simulink model "RobotSim"  (R2013a)
settings: Solver=ode45  StartTime=0.0  StopTime=5.00  FixedStep=0.01  MaxStep=0.02  MinStep=1e-16  RelTol=1e-3
values from neighbouring files (symbols this model uses):
  alpha_p = constr.alpha_p    [ConstrGui.m]    (also in RunSim.m = constrData(1).alpha_p; optimiseConstraint.m = [alpha_ends(:,1:2), alpha_p_infix, alpha_ends(:,3:4)])
  ground = [-realmax, 0 ... (first row only)    [RunSim.m]    (also in runSim2.m)
  nom_torque = [constrData.th_base; u_nom]    [RunSim.m]
  org = endSwingFoot(q(:,end),org)    [RunSim.m]    (also in runSim2.m = [0, 0])
  q_0 = q_0'    [RunSim.m]
  qd_0 = qd_0'    [RunSim.m]    (also in periodic_qd0.m = [2*pi; pi])
  theta_p = constr.theta_p    [ConstrGui.m]    (also in RunSim.m = constrData(1).theta_p; optimiseConstraint.m = linspace(theta_ends(1), theta_ends(2), degree+1))
settings Model: CovHTMLOptions=-sRT=1 -aTS=1 -bRG=1 -bTC=1 -hTR=0 -nFC=0 -scm=1 -bcm=1 -xEv=0  Creator=yak  LastModifiedBy=yak
settings SolverCC: MaxConsecutiveMinStep=10
settings DataIOCC: LimitDataPoints=off  OutputOption=SpecifiedOutputTimes  OutputTimes=0:0.01:(timeleft-0.01)
settings DebuggingCC: DiscreteInheritContinuousMsg=none  MultiTaskDSMMsg=warning  MultiTaskCondExecSysMsg=none  FcnCallInpInsideContextMsg=EnableAllAsWarning  StrictBusMsg=None
settings RTWCC: IncludeERTFirstTime=on

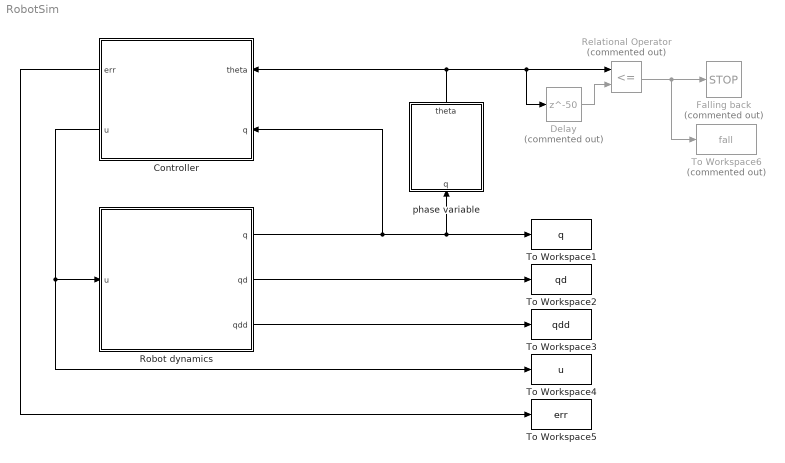
== system RobotSim ==
  Controller : Subsystem
  Delay : Delay  Commented=on  DelayLength=50  InitialCondition=-100  SampleTime=0.01
  Falling back : Stop  Commented=on
  Relational Operator : RelationalOperator  Commented=on  Operator=<=  OutDataTypeStr=boolean  ZeroCross=off
  Robot dynamics : Subsystem
  To Workspace1 : ToWorkspace  VariableName=q  SampleTime=-1
  To Workspace2 : ToWorkspace  VariableName=qd  SampleTime=-1
  To Workspace3 : ToWorkspace  VariableName=qdd  SampleTime=-1
  To Workspace4 : ToWorkspace  VariableName=u  SampleTime=-1
  To Workspace5 : ToWorkspace  VariableName=err  SampleTime=-1
  To Workspace6 : ToWorkspace  Commented=on  VariableName=fall  SampleTime=-1
      settings: MaxDataPoints=1
  phase variable : MATLAB Function  TreatAsAtomicUnit=on
  wires:
  Controller/2(u) -> Robot dynamics/1(u), To Workspace4/1
  Robot dynamics/1(q) -> Controller/2(q), To Workspace1/1, phase variable/1(q)
  Relational Operator/1 -> To Workspace6/1, Falling back/1
  phase variable/1(theta) -> Controller/1(theta), Delay/1, Relational Operator/1
  Robot dynamics/2(qd) -> To Workspace2/1
  Robot dynamics/3(qdd) -> To Workspace3/1
  Controller/1(err) -> To Workspace5/1
  Delay/1 -> Relational Operator/2

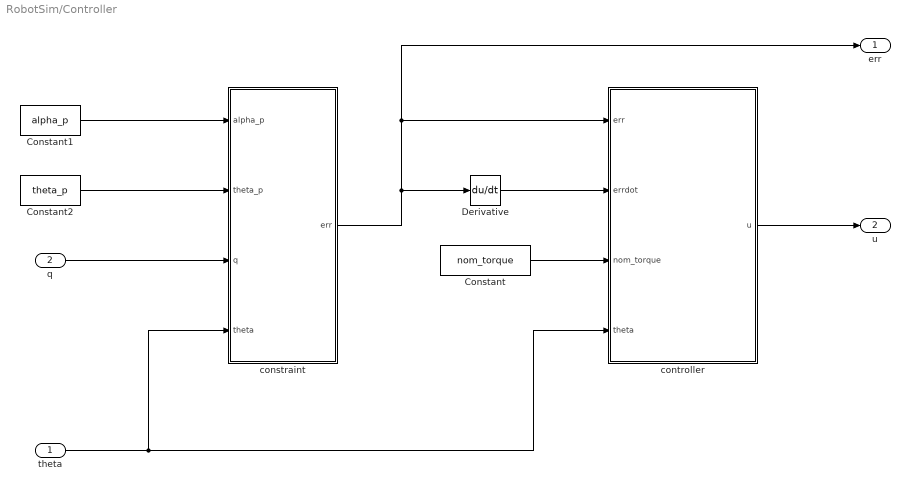
== system RobotSim/Controller ==
  theta : Inport
  q : Inport  Port=2
  Constant : Constant  Value=nom_torque
  Constant1 : Constant  Value=alpha_p  VectorParams1D=off
  Constant2 : Constant  Value=theta_p  VectorParams1D=off
  Derivative : Derivative
  constraint : MATLAB Function  TreatAsAtomicUnit=on
  controller : MATLAB Function  TreatAsAtomicUnit=on
  err : Outport
  u : Outport  Port=2
  wires:
  Constant/1 -> controller/3(nom_torque)
  Constant1/1 -> constraint/1(alpha_p)
  Constant2/1 -> constraint/2(theta_p)
  theta/1 -> controller/4(theta), constraint/4(theta)
  constraint/1(err) -> err/1, controller/1(err), Derivative/1
  Derivative/1 -> controller/2(errdot)
  q/1 -> constraint/3(q)
  controller/1(u) -> u/1

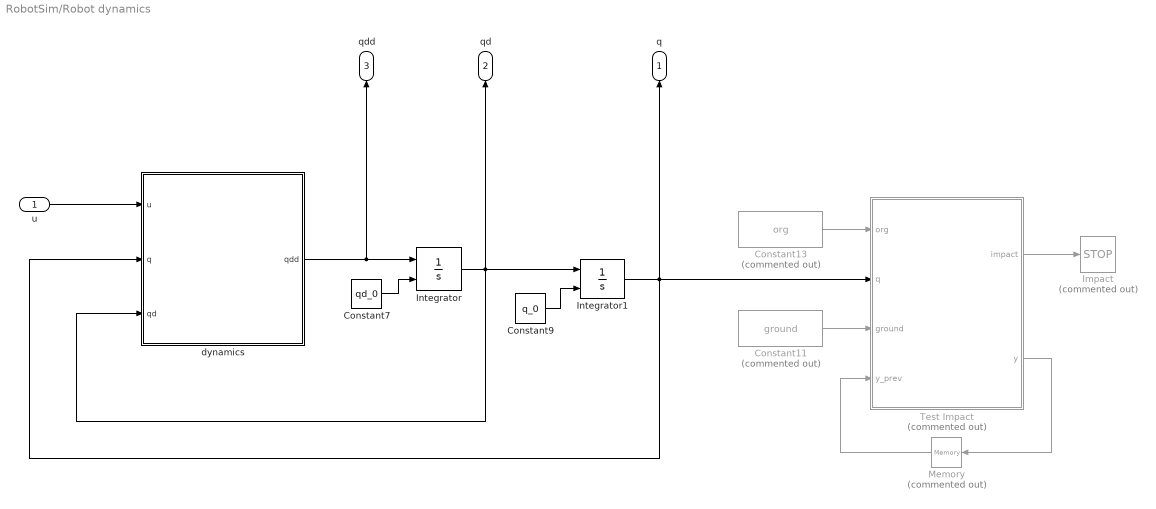
== system RobotSim/Robot dynamics ==
  u : Inport
  Constant11 : Constant  Commented=on  Value=ground  VectorParams1D=off
  Constant13 : Constant  Commented=on  Value=org  VectorParams1D=off
  Constant7 : Constant  Value=qd_0
  Constant9 : Constant  Value=q_0
  Impact : Stop  Commented=on
  Integrator : Integrator  InitialConditionSource=external
  Integrator1 : Integrator  InitialConditionSource=external
  Memory : Memory  Commented=on
  Test Impact : MATLAB Function  Commented=on  TreatAsAtomicUnit=on
  dynamics : MATLAB Function  TreatAsAtomicUnit=on
  q : Outport
  qd : Outport  Port=2
  qdd : Outport  Port=3
  wires:
  dynamics/1(qdd) -> qdd/1, Integrator/1
  Integrator/1 -> dynamics/3(qd), qd/1, Integrator1/1
  Integrator1/1 -> dynamics/2(q), q/1, Test Impact/2(q)
  Constant7/1 -> Integrator/2
  Constant9/1 -> Integrator1/2
  Test Impact/1(impact) -> Impact/1
  Constant11/1 -> Test Impact/3(ground)
  Test Impact/2(y) -> Memory/1
  Memory/1 -> Test Impact/4(y_prev)
  u/1 -> dynamics/1(u)
  Constant13/1 -> Test Impact/1(org)

== matlab function RobotSim/Robot dynamics/dynamics ==
  data: u input; qdd output; q input; qd input
function qdd = dynamics(u, q, qd)
%#codegen

[M, C, G, B] = dynMatrices(q,qd);

qdd = M\(B*u - C*qd - G);

end

== matlab function RobotSim/Robot dynamics/Test Impact ==
  data: org input; q input; ground input; impact output; y_prev input; y output
function [impact, y] = ...
    isImpact(org, q, ground, y_prev)
%#codegen

impact = false;
y=0;
height=0;

% Impact when the foot descends onto the ground after it has passed the
% midpoint of the swing phase.

% Calculate x and y position of foot.
p2 = endSwingFoot(q, org);

% Find height of ground underneath foot.
ind = find(p2(1)>ground(:,1), 1, 'last');
height = ground(ind,2);
height = height(1);
y = p2(2);

% Impact only if on falling edge and if stance leg is behind swing leg.
if y <= height && y_prev > height && ~scuff(q)
    impact = true;
end

end

== matlab function RobotSim/phase variable ==
  data: theta output; q input
function theta = phasevariable(q)
%#codegen

theta = phasevar(q);
end

== matlab function RobotSim/Controller/constraint ==
  data: alpha_p input; theta_p input; q input; theta input; err output
function err = constr(alpha_p, theta_p, q, theta)
%#codegen

% Calculate desired q
q_des = bezConstraint(theta_p, alpha_p, theta);

% Calculate error of actuated coordinate(s)
err = actuated(q_des-q);
% Ensure error is within 1 rotation
err = mod(err, 2*pi);   
% Ensure error is in the range [-pi pi]
err(err>pi) = err(err>pi) - 2*pi;
err(err<-pi) = err(err<-pi) + 2*pi;
end

== matlab function RobotSim/Controller/controller ==
  data: err input; errdot input; nom_torque input; theta input; u output
function u = controller(err, errdot, nom_torque, theta)
%#codegen

%% Feed-forward Zero Dynamics
% Linearly interpolate from pre-computed values.
i = find(theta >= nom_torque(1,:), 1, 'last');
if isempty(i)
    u = zeros(size(err));
else 
    i = i(1);
    if i < size(nom_torque,2)
        ths = nom_torque(1,i:i+1);
        us = nom_torque(2:end,i:i+1);
        u = (us(:,2)-us(:,1))/(ths(2)-ths(1))*(theta-ths(1)) + us(:,1);
    else
        u = zeros(size(err));
    end
end
u = 0;

%% Simple PD feedback controller
% This is used to correct any disturbance from the zero dynamics
K_p = 1000;
K_d = 100;

u = u + K_p*err + K_d*errdot;
end
